simulink model "Casadi_Custom_Driver"  (R2016b)
settings: Solver=FixedStepDiscrete  StartTime=0.0  StopTime=inf  FixedStep=0.01  RelTol=1e-3  EnableMultiTasking=on
undefined symbols (not defined in the file): dimensionsFactor, DiscIntNeverNeededParam, vehicle_name, VehicleRoadInfoStructSize
libraries: simulink x39, SCANeR_API x36
(part 1 of 3)
settings Model: SimulationMode=accelerator  TunableVars=vehicle_name  TunableVarsStorageClass=ExportedGlobal  Creator=a192819  LastModifiedBy=z041288
settings DataIOCC: LimitDataPoints=on  SaveFormat=Array  SaveOutput=off  SignalLogging=off  DSMLogging=off  SaveTime=off  SignalLoggingName=virtual_driver
settings DebuggingCC: SignalInfNanChecking=warning  UnderspecifiedInitializationDetection=Classic  MergeDetectMultiDrivingBlocksExec=none  SolverPrmCheckMsg=warning  SFUnexpectedBacktrackingDiag=warning  SFNoUnconditionalDefaultTransitionDiag=warning  SFExecutionAtInitializationDiag=none
settings HardwareCC: ProdBitPerPointer=32  ProdBitPerSizeT=32  ProdBitPerPtrDiffT=32  ProdLargestAtomicFloat=None  ProdIntDivRoundTo=Undefined  ProdEndianess=Unspecified  ProdWordSize=32  ProdHWDeviceType=32-bit Generic
settings ModelReferenceCC: PropagateSignalLabelsOutOfModel=off
settings RTWCC: SystemTargetFile=grt_scanerapi.tlc  TemplateMakefile=grt_scanerapi_vc.tmf  Description=SCANeR API Real-Time Target  CustomSource=ReadConfig.c  CustomInitializer=ReadConfig();
settings STFCustomTargetCC: MatFileLogging=on  SystemTargetFile=grt_scanerapi.tlc
settings GRTTargetCC: TargetLangStandard=C89/C90 (ANSI)  ParMdlRefBuildCompliant=off  CompOptLevelCompliant=off  ConcurrentExecutionCompliant=off  CombineOutputUpdateFcns=off  CPPClassGenCompliant=off  GRTInterface=on  UseToolchainInfoCompliant=off
settings ConfigComp: CovMetricSettings=dw  CovHtmlReporting=on  CovSaveCumulativeToWorkspaceVar=on  CovSaveSingleToWorkspaceVar=on  CovExternalEMLEnable=off

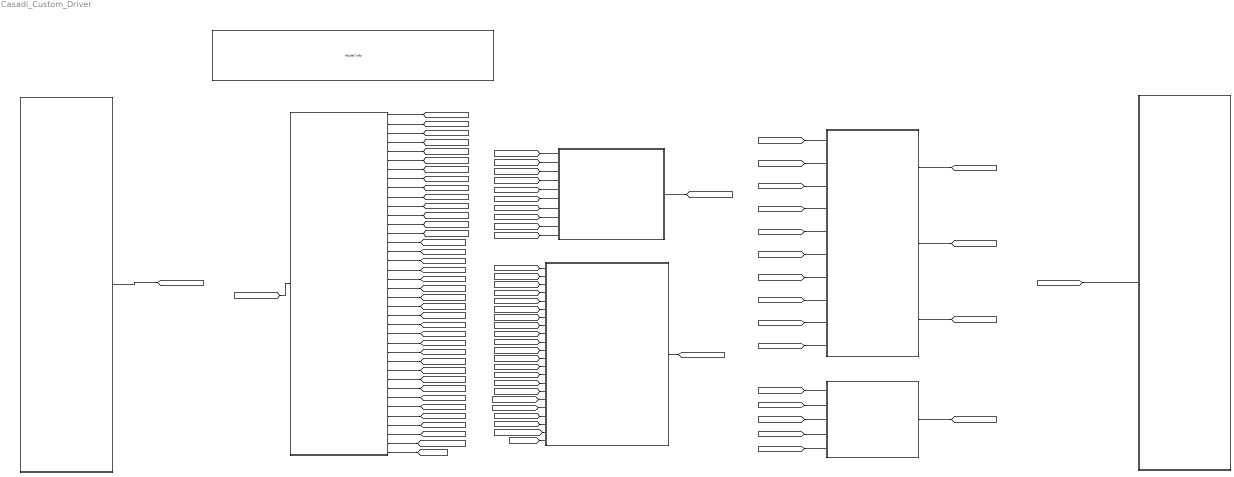
== system Casadi_Custom_Driver ==
  note: From SCANeR
  note: To SCANeR
  note: Arbitration
  note: Lateral control
  note: Longitudinal control
  note: InputSignalsManagement
  note: Custom_Driver_Architecture
  note: Custom_Driver_Environnement
  note: OutputSignalsManagement
  From Scaner : Subsystem
  Input_Signals_Management : Subsystem
  Model Info1 : simulink/Model-Wide Utilities/Model Info  Frame=on  DisplayStringWithTags=|  HorizontalTextAlignment=Left  LeftAlignmentValue=0.02  SourceBlockDiagram=Casadi_Custom_Driver  TagMaxNumber=20
      | CUSTOM DRIVER FOR SCANER
      | 
      | Developed and maintained by :
      |    - Hamid Dahmani (DEA-TDV3) (2017 => Oct. 2018)
      |    - Eric Cabrol (DEA-TDS3) (Oct. 2018 => 2020)
      |    - Eric Cabrol (DEA-TDS3) & Adithya Rajasekaran (RNTBCI) (2020 => 2021)
      |    - Eric Cabrol (DEA-TDS3), KATRE Varun-Dattakumar (RNTBCI) & Soumaya DKHEILA (DEA-TDV3) (2021 => Present)
      | 
      | Version: %<ModelVersion>
      | Last update by: %<LastModifiedBy>, Date: %<LastModificationDate>.
  Output_Signals_Management : Subsystem
  To Scaner : Subsystem
  driver manager : Subsystem
  lateral control : Subsystem
  longitudinal control : Subsystem
  wires:
  From Scaner/1(FromSCANeR_O) -> [FromSCANeR_I]
  [ToSCANeR_O] -> To Scaner/1(ToSCANeR_I)
  [FromSCANeR_I] -> Input_Signals_Management/1(From_SCANeR_I)
  Input_Signals_Management/2(vehicleHeading) -> [vehicleHeading]
  Input_Signals_Management/3(COG_Y) -> [COG_Y]
  Input_Signals_Management/4(currentSpeed) -> [currentSpeed]
  Input_Signals_Management/5(yawRate) -> [yawRate]
  Input_Signals_Management/6(currentAccel) -> [currentAcceleration]
  Input_Signals_Management/7(SteeringWheelAngle) -> [SteeringWheelAngle]
  Input_Signals_Management/8(gearEngaged) -> [gearEngaged]
  Input_Signals_Management/9(roadGap) -> [roadGap]
  Input_Signals_Management/10(roadAngle) -> [roadAngle]
  Input_Signals_Management/12(roadGapOffset) -> [roadGapOffset]
  Input_Signals_Management/11(laneGap) -> [laneGap]
  Input_Signals_Management/13(obligatorySpeed) -> [obligatorySpeed]
  Input_Signals_Management/14(obligatorySpeedState) -> [obligatorySpeedState]
  Input_Signals_Management/19(timeToReactShift) -> [timeToReactShift]
  Input_Signals_Management/16(obligatoryAccelerationState) -> [obligatoryAccelerationState]
  Input_Signals_Management/15(obligatoryAcceleration) -> [obligatoryAcceleration]
  Input_Signals_Management/17(shiftType) -> [shiftType]
  Input_Signals_Management/18(shiftValue) -> [shiftValue]
  Input_Signals_Management/27(ManualBrakeforceActivate) -> [ManualBrakeforceActivate]
  Input_Signals_Management/29(APK_Steering) -> [APK_Steering]
  Input_Signals_Management/30(clothoidAngle) -> [ClothoidAngle]
  Input_Signals_Management/28(ManualAccelActivate) -> [ManualAccelActivate]
  Input_Signals_Management/20(ManualBrakeForce) -> [ManualBrakeForce]
  Input_Signals_Management/21(ManualBrake) -> [ManualBrake]
  Input_Signals_Management/22(ManualAccel) -> [ManualAccel]
  Input_Signals_Management/25(APK_steeringActivate) -> [APK_steeringActivate]
  Input_Signals_Management/23(WantedLateralShiftSpeed) -> [WantedLateralShiftSpeed]
  Input_Signals_Management/26(ManualBrakeActivate) -> [ManualBrakeActivate]
  Input_Signals_Management/24(SteeringTorqueOrder) -> [SteeringTorqueOrder]
  Input_Signals_Management/31(SteeringTorqueRequest) -> [SteeringTorqueRequest]
  Input_Signals_Management/34(RadiusCurvatureSetPoint) -> [RadiusCurvatureSetPoint]
  Input_Signals_Management/35(VehiculeWantedGearBox) -> [VehiculeWantedGearBox]
  Input_Signals_Management/33(LaneCurvature) -> [LaneCurvature]
  Input_Signals_Management/32(DriverStatus) -> [DriverStatus]
  Input_Signals_Management/1(SCANeR_State) -> [SCANeR_State]
  [laneGap] -> lateral control/1(Lane_gap_m)
  [LaneCurvature] -> lateral control/2(RoadCurvature_pm)
  [currentSpeed] -> lateral control/3(Vh_Speed_m/s)
  [shiftValue] -> lateral control/4(Shift_Value)
  [timeToReactShift] -> lateral control/5(Shift_time_s)
  [roadAngle] -> lateral control/6(Road_Angle_rad)
  [vehicleHeading] -> lateral control/7(Vehicle_Heading_rad)
  [SCANeR_State] -> lateral control/8(SCANeR_State)
  [shiftType] -> lateral control/10(Shift_Type_1Met_0Lan)
  [roadGap] -> lateral control/11(Road_Gap_m)
  [roadGapOffset] -> lateral control/12(Road_Gap_Offset_m)
  [gearEngaged] -> lateral control/13(SCANeR_gearEngaged)
  [WantedLateralShiftSpeed] -> lateral control/14(wantedLateralShiftSpeed)
  [SteeringWheelAngle] -> lateral control/15(SW_angle_IN)
  [yawRate] -> lateral control/16(yaw rate)
  [ClothoidAngle] -> lateral control/17(clothoid_tangent_angle)
  [RadiusCurvatureSetPoint] -> lateral control/18(clothoid_flag)
  [COG_Y] -> lateral control/19(COG_Y)
  [DriverStatus] -> driver manager/2(SCANeR_DriverStatus)
  [ManualAccel] -> driver manager/3(Manual_accel_%)
  [ManualAccelActivate] -> driver manager/4(Manual_accel_%_activate)
  [ManualBrake] -> driver manager/5(Manual_brake_%)
  [ManualBrakeActivate] -> driver manager/6(Manual_brake_%_activate)
  [APK_Steering] -> driver manager/7(APK_steering_rad)
  [APK_steeringActivate] -> driver manager/8(APK_steering_rad_Activate)
  [SCANeR_State] -> driver manager/9(SCANeR_State)
  longitudinal control/1(Driver_Action_to_SCANeR_Longi) -> [Driver_Action_to_SCANeR_Longi]
  [Driver_Action_to_SCANeR_Longi] -> driver manager/1(Driver_Action_to_SCANeR_Long)
  lateral control/1(Driver_Action_to_SCANeR_Lat) -> [Driver_Action_to_SCANeR_Lat]
  [Driver_Action_to_SCANeR_Lat] -> driver manager/10(Driver_Action_to_SCANeR_Lat)
  driver manager/2(SCANeR_DriverStatus_Out) -> [DriverStatus_O]
  [DriverStatus_O] -> lateral control/9(SCANeR_DriverStatus_Out)
  driver manager/1(Driver_Action_to_SCANeR_Longi_out) -> [Driver_Action_to_SCANeR_Longi_out]
  driver manager/3(Driver_Action_to_SCANeR_Lat_out) -> [Driver_Action_to_SCANeR_Lat_out]
  Output_Signals_Management/1(ToSCANeR_O) -> [ToSCANeR_O]
  [SteeringTorqueRequest] -> Output_Signals_Management/5(SteeringTorqueRequest)
  [SteeringTorqueOrder] -> Output_Signals_Management/4(SteeringTorqueOrder)
  [VehiculeWantedGearBox] -> Output_Signals_Management/3(VehiculeWantedGearBox)
  [Driver_Action_to_SCANeR_Longi_out] -> Output_Signals_Management/1(Driver_Action_to_SCANeR_Longi_out)
  [Driver_Action_to_SCANeR_Lat_out] -> Output_Signals_Management/2(Driver_Action_to_SCANeR_Lat_out)
  [obligatorySpeed] -> longitudinal control/1(Intended_Vehicle_Speed_[m/s])
  [obligatoryAcceleration] -> longitudinal control/4(Intended_Vehicle_accel_[m/s2])
  [obligatoryAccelerationState] -> longitudinal control/6(Accel_control_on)
  [SCANeR_State] -> longitudinal control/9(SCANeR_State)
  [ManualBrakeForce] -> longitudinal control/7(Manual_braking_N)
  [currentAcceleration] -> longitudinal control/5(Vehicle_accel_[m/s2])
  [currentSpeed] -> longitudinal control/2(Vehicle_Speed_[m/s])
  [ManualBrakeforceActivate] -> longitudinal control/8(Manual_braking_Switch)
  [DriverStatus_O] -> longitudinal control/10(SCANeR_DriverStatus_Out)
  [obligatorySpeedState] -> longitudinal control/3(Speed_control_on)
  Input_Signals_Management/36(Flag_detect_banking) -> [Flag_detect_banking]
  [Flag_detect_banking] -> lateral control/20(Flag_detect_banking)
  Input_Signals_Management/37(COG_X) -> [COG_X]
  Input_Signals_Management/38(current_lateral_speed) -> [current_lateral_speed]
  [current_lateral_speed] -> lateral control/22(measured_lateral_speed)
  [COG_X] -> lateral control/21(COG_X)

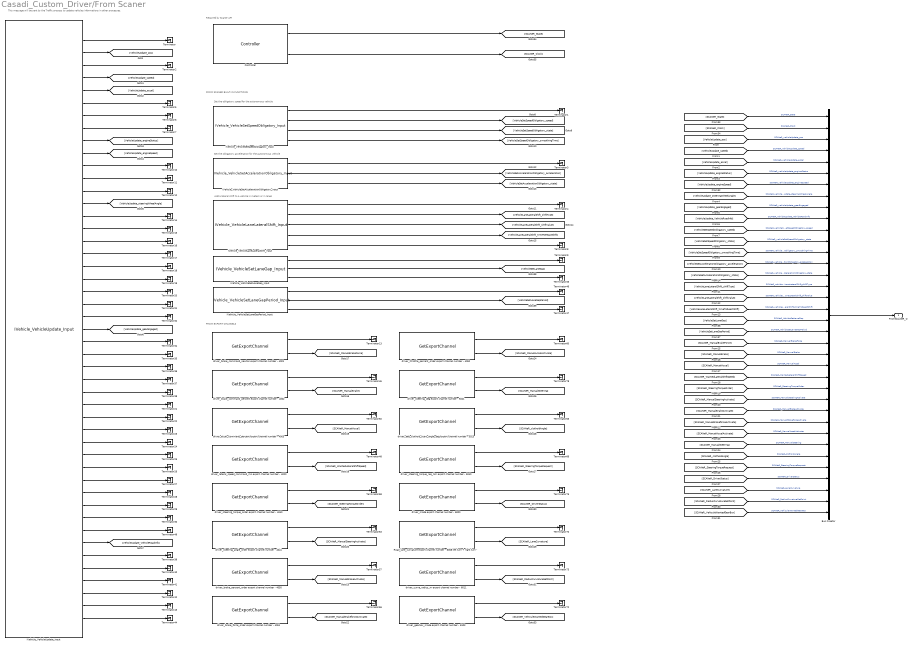
== system Casadi_Custom_Driver/From Scaner ==
  note: Set the obligatory speed for the autonomous vehicle
  note: Set the obligatory acceleration for the autonomous vehicle
  note: Add a lateral shift to a vehicle in meters or in lanes
  note: This message will be sent by the Traffic process to update vehicles informations in other processes.
  note: FROM EXPORT CHANNELS
  note: FROM SCANER BUILT-IN FUNCTIONS
  note: Required by Scaner API
  Bus Creator : BusCreator  Inputs='SCANeR_State','SCANeR_Clock','SCANeR_vehicleUpdate_pos','SCANeR_vehicleUpdate_speed','SCANeR_vehicleUpdate_accel','SCANeR_vehicleUpdate_engineStatus','SCANeR_vehicleUpdate_engineSpeed','SCANeR_vehicleUpdate_steeringWheelAngle','SCANeR_vehicleUpdate_gearEngaged','SCANeR_vehicleUpdate_VehicleRoadInfo','SCANeR_vehicleSetSpeedObligatory_speed','SCANeR_vehicleSetSpeedObligatory_state','SCANeR_vehicleSetSpeedObligatory_smoothingTime','SCANeR_vehicleSetAccelerationObligatory_acceleration','SCANeR_vehicleSetAccelerationObligatory_state','SCANeR_vehicleLaneLateralShift_shiftType','SCANeR_vehicleLaneLateralShift_shiftValue','SCANeR_vehicleLaneLateralShift_timeToReactShift','SCANeR_VehicleSetLaneGap','SCANeR_VehicleSetLaneGapPeriod','SCANeR_ManualBrakeForce','SCANeR_ManualBrake','SCANeR_ManualAccel','SCANeR_WantedLateralShiftSpeed','SCANeR_SteeringTorqueOrder','SCANeR_ManualSteeringActivate','SCANeR_ManualBrakeActivate','SCANeR_ManualBrakeforceActivate','SCANeR_ManualAccelActivate','SCANeR_ManualSteering','SCANeR_clothoidAngle','SCANeR_SteeringTorqueRequest','SCANeR_DriverStatus','SCANeR_LaneCurvature','SCANeR_RadiusCurvatureSetPoint','SCANeR_VehiculeWantedGearBox'  OutDataTypeStr=Bus: Bus_FromSCANeR
  Controller : SCANeR_API/Controller  Priority=1  Config='NEWCONFIG_Training'  ProcName='SIMULINK'  Frequency=-100  NetworkOutputFrequency=-100  TimeOut=300  IsSynchronized=on
  IVehicle_VehicleLaneLateralShift_Input : SCANeR_API/Network inputs/IVehicle/IVehicle_VehicleLaneLateralShift_Input  Priority=2  ev=off  vhlId=0
  IVehicle_VehicleSetAccelerationObligatory_Input : SCANeR_API/Network inputs/IVehicle/IVehicle_VehicleSetAccelerationObligatory_Input  Priority=2  ev=off  vhlId=0
  IVehicle_VehicleSetLaneGapPeriod_Input : SCANeR_API/Network inputs/IVehicle/IVehicle_VehicleSetLaneGapPeriod_Input  Priority=2  ev=off  vhlId=0
  IVehicle_VehicleSetLaneGap_Input : SCANeR_API/Network inputs/IVehicle/IVehicle_VehicleSetLaneGap_Input  Priority=2  ev=off  vhlId=0
  IVehicle_VehicleSetSpeedObligatory_Input : SCANeR_API/Network inputs/IVehicle/IVehicle_VehicleSetSpeedObligatory_Input  Priority=2  ev=off  vhlId=0
  IVehicle_VehicleUpdate_Input : SCANeR_API/Network inputs/IVehicle/IVehicle_VehicleUpdate_Input  Priority=2  ev=off  vhlId=0
  Road_lane_curvature export channel number - 6008 left turn + right turn - : SCANeR_API/GetExportChannel  Priority=0  ExportChannelCategory='system'  ExportChannelName='Road_lane_curvature'  VehicleId=-1
  Terminator{,1..50,53,56..58,60,63,66,70,72..73,75,78} (63 alike) : Terminator
  driver_accel_command_percent export channel number - 4003 : SCANeR_API/GetExportChannel  Priority=0  ExportChannelCategory='system'  ExportChannelName='driver_accel_command_percent'  VehicleId=-1
  driver_aeb_clothoid_start_angle_deg export channel number - 5023 : SCANeR_API/GetExportChannel  Priority=0  ExportChannelCategory='system'  ExportChannelName='driver_aeb_clothoid_start_angle_deg'  VehicleId=-1
  driver_brake_command_newton export channel number - 4001 : SCANeR_API/GetExportChannel  Priority=0  ExportChannelCategory='system'  ExportChannelName='driver_brake_command_newton'  VehicleId=-1
  driver_brake_command_percent export channel number - 4002 : SCANeR_API/GetExportChannel  Priority=0  ExportChannelCategory='system'  ExportChannelName='driver_brake_command_percent'  VehicleId=-1
  driver_brake_force_order export channel number - 4051 : SCANeR_API/GetExportChannel  Priority=0  ExportChannelCategory='system'  ExportChannelName='driver_brake_force_order'  VehicleId=-1
  driver_brake_percent_order export channel number - 4050 : SCANeR_API/GetExportChannel  Priority=0  ExportChannelCategory='system'  ExportChannelName='driver_brake_percent_order'  VehicleId=-1
  driver_curve_radius_m export channel number - 6011 : SCANeR_API/GetExportChannel  Priority=0  ExportChannelCategory='system'  ExportChannelName='driver_curve_radius_m'  VehicleId=-1
  driver_gearbox_mode export channel number - 6103 : SCANeR_API/GetExportChannel  Priority=0  ExportChannelCategory='system'  ExportChannelName='driver_gearbox_mode'  VehicleId=-1
  driver_lateral_speed_command_ms export channel number - 4020 : SCANeR_API/GetExportChannel  Priority=0  ExportChannelCategory='system'  ExportChannelName='driver_lateral_speed_command_ms'  VehicleId=-1
  driver_mode export channel number - 6000 : SCANeR_API/GetExportChannel  Priority=0  ExportChannelCategory='system'  ExportChannelName='driver_mode'  VehicleId=-1
  driver_steering_angle_order export channel number - 4041 : SCANeR_API/GetExportChannel  Priority=0  ExportChannelCategory='system'  ExportChannelName='driver_steering_angle_order'  VehicleId=-1
  driver_steering_deg export channel number - 5021 : SCANeR_API/GetExportChannel  Priority=0  ExportChannelCategory='system'  ExportChannelName='driver_steering_deg'  VehicleId=-1
  driver_steering_torque_order export channel number - 4040 : SCANeR_API/GetExportChannel  Priority=0  ExportChannelCategory='system'  ExportChannelName='driver_steering_torque_order'  VehicleId=-1
  driver_steering_torque_req_Nm export channel number - 5040 : SCANeR_API/GetExportChannel  Priority=0  ExportChannelCategory='system'  ExportChannelName='driver_steering_torque_req_Nm'  VehicleId=-1
  driver_throttle_percent_order export channel number - 4052 : SCANeR_API/GetExportChannel  Priority=0  ExportChannelCategory='system'  ExportChannelName='driver_throttle_percent_order'  VehicleId=-1
  FromSCANeR_O : Outport  OutDataTypeStr=Bus: Bus_FromSCANeR
      settings: AttributesFormatString=%<OutDataTypeStr>
  wires:
  IVehicle_VehicleUpdate_Input/1 -> Terminator/1
  IVehicle_VehicleUpdate_Input/2 -> [VehicleUpdate_pos]
  IVehicle_VehicleUpdate_Input/3 -> Terminator2/1
  IVehicle_VehicleUpdate_Input/4 -> [VehicleUpdate_speed]
  IVehicle_VehicleUpdate_Input/5 -> [VehicleUpdate_accel]
  IVehicle_VehicleUpdate_Input/6 -> Terminator5/1
  IVehicle_VehicleUpdate_Input/7 -> Terminator6/1
  IVehicle_VehicleUpdate_Input/8 -> Terminator7/1
  IVehicle_VehicleUpdate_Input/9 -> [VehicleUpdate_engineStatus]
  IVehicle_VehicleUpdate_Input/10 -> [VehicleUpdate_engineSpeed]
  IVehicle_VehicleUpdate_Input/11 -> Terminator10/1
  IVehicle_VehicleUpdate_Input/12 -> Terminator11/1
  IVehicle_VehicleUpdate_Input/13 -> Terminator12/1
  IVehicle_VehicleUpdate_Input/14 -> [VehicleUpdate_steeringWheelAngle]
  IVehicle_VehicleUpdate_Input/15 -> Terminator14/1
  IVehicle_VehicleUpdate_Input/16 -> Terminator15/1
  IVehicle_VehicleUpdate_Input/17 -> Terminator16/1
  IVehicle_VehicleUpdate_Input/18 -> Terminator17/1
  IVehicle_VehicleUpdate_Input/19 -> Terminator18/1
  IVehicle_VehicleUpdate_Input/20 -> Terminator19/1
  IVehicle_VehicleUpdate_Input/21 -> Terminator20/1
  IVehicle_VehicleUpdate_Input/22 -> Terminator31/1
  IVehicle_VehicleUpdate_Input/23 -> Terminator32/1
  IVehicle_VehicleUpdate_Input/24 -> [VehicleUpdate_gearEngaged]
  IVehicle_VehicleUpdate_Input/25 -> Terminator34/1
  IVehicle_VehicleUpdate_Input/26 -> Terminator35/1
  IVehicle_VehicleUpdate_Input/27 -> Terminator36/1
  IVehicle_VehicleUpdate_Input/28 -> Terminator37/1
  IVehicle_VehicleUpdate_Input/29 -> Terminator38/1
  IVehicle_VehicleUpdate_Input/30 -> Terminator21/1
  IVehicle_VehicleUpdate_Input/31 -> Terminator22/1
  IVehicle_VehicleUpdate_Input/32 -> Terminator23/1
  IVehicle_VehicleUpdate_Input/34 -> Terminator25/1
  IVehicle_VehicleUpdate_Input/35 -> Terminator26/1
  IVehicle_VehicleUpdate_Input/36 -> Terminator27/1
  IVehicle_VehicleUpdate_Input/37 -> Terminator28/1
  IVehicle_VehicleUpdate_Input/38 -> Terminator29/1
  IVehicle_VehicleUpdate_Input/39 -> Terminator30/1
  IVehicle_VehicleUpdate_Input/40 -> Terminator49/1
  IVehicle_VehicleUpdate_Input/41 -> [VehicleUpdate_VehicleRoadInfo]
  IVehicle_VehicleUpdate_Input/42 -> Terminator39/1
  IVehicle_VehicleUpdate_Input/43 -> Terminator40/1
  IVehicle_VehicleUpdate_Input/44 -> Terminator41/1
  IVehicle_VehicleUpdate_Input/45 -> Terminator42/1
  IVehicle_VehicleUpdate_Input/46 -> Terminator43/1
  IVehicle_VehicleUpdate_Input/47 -> Terminator44/1
  IVehicle_VehicleUpdate_Input/33 -> Terminator24/1
  IVehicle_VehicleSetSpeedObligatory_Input/1 -> Terminator1/1
  IVehicle_VehicleSetSpeedObligatory_Input/2 -> [VehicleSetSpeedObligatory_speed]
  IVehicle_VehicleSetSpeedObligatory_Input/4 -> [VehicleSetSpeedObligatory_smoothingTime]
  IVehicle_VehicleSetSpeedObligatory_Input/3 -> [VehicleSetSpeedObligatory_state]
  IVehicle_VehicleSetAccelerationObligatory_Input/1 -> Terminator3/1
  IVehicle_VehicleLaneLateralShift_Input/1 -> Terminator4/1
  IVehicle_VehicleLaneLateralShift_Input/5 -> Terminator8/1
  IVehicle_VehicleSetAccelerationObligatory_Input/2 -> [VehicleSetAccelerationObligatory_acceleration]
  IVehicle_VehicleSetAccelerationObligatory_Input/3 -> [VehicleSetAccelerationObligatory_state]
  IVehicle_VehicleLaneLateralShift_Input/2 -> [VehicleLaneLateralShift_shiftType]
  IVehicle_VehicleLaneLateralShift_Input/3 -> [VehicleLaneLateralShift_shiftValue]
  IVehicle_VehicleLaneLateralShift_Input/4 -> [VehicleLaneLateralShift_timeToReactShift]
  driver_brake_command_newton export channel number - 4001/1 -> Terminator13/1
  driver_brake_command_newton export channel number - 4001/2 -> [SCANeR_ManualBrakeForce]
  driver_brake_command_percent export channel number - 4002/1 -> Terminator45/1
  driver_brake_command_percent export channel number - 4002/2 -> [SCANeR_ManualBrake]
  driver_accel_command_percent export channel number - 4003/1 -> Terminator50/1
  driver_accel_command_percent export channel number - 4003/2 -> [SCANeR_ManualAccel]
  driver_lateral_speed_command_ms export channel number - 4020/1 -> Terminator48/1
  driver_lateral_speed_command_ms export channel number - 4020/2 -> [SCANeR_WantedLateralShiftSpeed]
  driver_steering_torque_order export channel number - 4040/1 -> Terminator58/1
  driver_steering_torque_order export channel number - 4040/2 -> [SCANeR_SteeringTorqueOrder]
  driver_steering_angle_order export channel number - 4041/1 -> Terminator53/1
  driver_steering_angle_order export channel number - 4041/2 -> [SCANeR_ManualSteeringActivate]
  driver_brake_percent_order export channel number - 4050/1 -> Terminator57/1
  driver_brake_percent_order export channel number - 4050/2 -> [SCANeR_ManualBrakeActivate]
  driver_brake_force_order export channel number - 4051/1 -> Terminator56/1
  driver_brake_force_order export channel number - 4051/2 -> [SCANeR_ManualBrakeforceActivate]
  driver_throttle_percent_order export channel number - 4052/1 -> Terminator60/1
  driver_throttle_percent_order export channel number - 4052/2 -> [SCANeR_ManualAccelActivate]
  driver_steering_deg export channel number - 5021/1 -> Terminator78/1
  driver_steering_deg export channel number - 5021/2 -> [SCANeR_ManualSteering]
  driver_aeb_clothoid_start_angle_deg export channel number - 5023/1 -> Terminator63/1
  driver_aeb_clothoid_start_angle_deg export channel number - 5023/2 -> [SCANeR_clothoidAngle]
  driver_steering_torque_req_Nm export channel number - 5040/1 -> Terminator66/1
  driver_steering_torque_req_Nm export channel number - 5040/2 -> [SCANeR_SteeringTorqueRequest]
  driver_mode export channel number - 6000/1 -> Terminator75/1
  driver_mode export channel number - 6000/2 -> [SCANeR_DriverStatus]
  Road_lane_curvature export channel number - 6008 left turn + right turn -/1 -> Terminator70/1
  Road_lane_curvature export channel number - 6008 left turn + right turn -/2 -> [SCANeR_LaneCurvature]
  driver_curve_radius_m export channel number - 6011/1 -> Terminator73/1
  driver_gearbox_mode export channel number - 6103/1 -> Terminator72/1
  driver_curve_radius_m export channel number - 6011/2 -> [SCANeR_RadiusCurvatureSetPoint]
  driver_gearbox_mode export channel number - 6103/2 -> [SCANeR_VehiculeWantedGearBox]
  [VehicleUpdate_pos] -> Bus Creator/3  "SCANeR_vehicleUpdate_pos"
  [VehicleUpdate_engineSpeed] -> Bus Creator/7  "SCANeR_vehicleUpdate_engineSpeed"
  [VehicleUpdate_engineStatus] -> Bus Creator/6  "SCANeR_vehicleUpdate_engineStatus"
  [VehicleUpdate_accel] -> Bus Creator/5  "SCANeR_vehicleUpdate_accel"
  [VehicleUpdate_speed] -> Bus Creator/4  "SCANeR_vehicleUpdate_speed"
  [VehicleUpdate_steeringWheelAngle] -> Bus Creator/8  "SCANeR_vehicleUpdate_steeringWheelAngle"
  [VehicleUpdate_gearEngaged] -> Bus Creator/9  "SCANeR_vehicleUpdate_gearEngaged"
  [VehicleUpdate_VehicleRoadInfo] -> Bus Creator/10  "SCANeR_vehicleUpdate_VehicleRoadInfo"
  [VehicleSetSpeedObligatory_speed] -> Bus Creator/11  "SCANeR_vehicleSetSpeedObligatory_speed"
  [VehicleSetSpeedObligatory_state] -> Bus Creator/12  "SCANeR_vehicleSetSpeedObligatory_state"
  [VehicleSetSpeedObligatory_smoothingTime] -> Bus Creator/13  "SCANeR_vehicleSetSpeedObligatory_smoothingTime"
  [VehicleSetAccelerationObligatory_acceleration] -> Bus Creator/14  "SCANeR_vehicleSetAccelerationObligatory_acceleration"
  [VehicleSetAccelerationObligatory_state] -> Bus Creator/15  "SCANeR_vehicleSetAccelerationObligatory_state"
  [VehicleLaneLateralShift_shiftType] -> Bus Creator/16  "SCANeR_vehicleLaneLateralShift_shiftType"
  [VehicleLaneLateralShift_shiftValue] -> Bus Creator/17  "SCANeR_vehicleLaneLateralShift_shiftValue"
  [VehicleLaneLateralShift_timeToReactShift] -> Bus Creator/18  "SCANeR_vehicleLaneLateralShift_timeToReactShift"
  Controller/1 -> [SCANeR_State]
  Controller/2 -> [SCANeR_Clock]
  [SCANeR_Clock] -> Bus Creator/2  "SCANeR_Clock"
  [SCANeR_State] -> Bus Creator/1  "SCANeR_State"
  Bus Creator/1 -> FromSCANeR_O/1
  IVehicle_VehicleSetLaneGap_Input/2 -> [VehicleSetLaneGap]
  IVehicle_VehicleSetLaneGapPeriod_Input/2 -> [VehicleSetLaneGapPeriod]
  IVehicle_VehicleSetLaneGap_Input/1 -> Terminator9/1
  IVehicle_VehicleSetLaneGap_Input/3 -> Terminator33/1
  IVehicle_VehicleSetLaneGapPeriod_Input/1 -> Terminator46/1
  IVehicle_VehicleSetLaneGapPeriod_Input/3 -> Terminator47/1
  [SCANeR_ManualBrakeForce] -> Bus Creator/21  "SCANeR_ManualBrakeForce"
  [SCANeR_ManualBrake] -> Bus Creator/22  "SCANeR_ManualBrake"
  [SCANeR_ManualAccel] -> Bus Creator/23  "SCANeR_ManualAccel"
  [SCANeR_WantedLateralShiftSpeed] -> Bus Creator/24  "SCANeR_WantedLateralShiftSpeed"
  [SCANeR_SteeringTorqueOrder] -> Bus Creator/25  "SCANeR_SteeringTorqueOrder"
  [SCANeR_ManualSteeringActivate] -> Bus Creator/26  "SCANeR_ManualSteeringActivate"
  [SCANeR_ManualBrakeActivate] -> Bus Creator/27  "SCANeR_ManualBrakeActivate"
  [SCANeR_ManualBrakeforceActivate] -> Bus Creator/28  "SCANeR_ManualBrakeforceActivate"
  [SCANeR_ManualAccelActivate] -> Bus Creator/29  "SCANeR_ManualAccelActivate"
  [SCANeR_ManualSteering] -> Bus Creator/30  "SCANeR_ManualSteering"
  [SCANeR_clothoidAngle] -> Bus Creator/31  "SCANeR_clothoidAngle"
  [SCANeR_SteeringTorqueRequest] -> Bus Creator/32  "SCANeR_SteeringTorqueRequest"
  [SCANeR_DriverStatus] -> Bus Creator/33  "SCANeR_DriverStatus"
  [SCANeR_LaneCurvature] -> Bus Creator/34  "SCANeR_LaneCurvature"
  [SCANeR_RadiusCurvatureSetPoint] -> Bus Creator/35  "SCANeR_RadiusCurvatureSetPoint"
  [SCANeR_VehiculeWantedGearBox] -> Bus Creator/36  "SCANeR_VehiculeWantedGearBox"
  [VehicleSetLaneGap] -> Bus Creator/19  "SCANeR_VehicleSetLaneGap"
  [VehicleSetLaneGapPeriod] -> Bus Creator/20  "SCANeR_VehicleSetLaneGapPeriod"

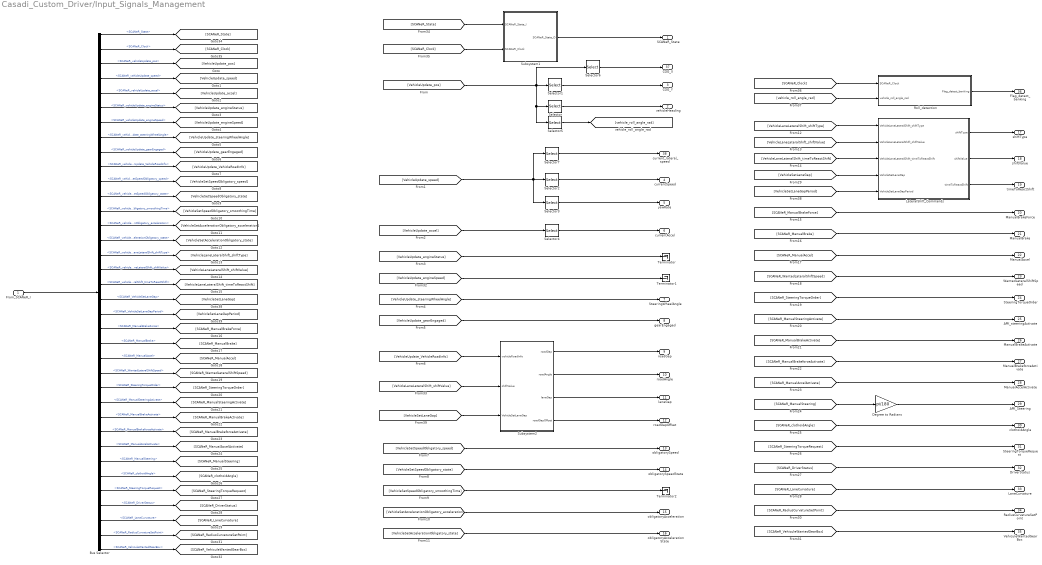
== system Casadi_Custom_Driver/Input_Signals_Management ==
  From_SCANeR_I : Inport  OutDataTypeStr=Bus: Bus_FromSCANeR
      settings: AttributesFormatString=%<OutDataTypeStr>
  Bus Selector : BusSelector  OutputSignals=SCANeR_State,SCANeR_Clock,SCANeR_vehicleUpdate_pos,SCANeR_vehicleUpdate_speed,SCANeR_vehicleUpdate_accel,SCANeR_vehicleUpdate_engineStatus,SCANeR_vehicleUpdate_engineSpeed,SCANeR_vehicleUpdate_steeringWheelAngle,SCANeR_vehicleUpdate_gearEngaged,SCANeR_vehicleUpdate_VehicleRoadInfo,SCANeR_vehicleSetSpeedObligatory_speed,SCANeR_vehicleSetSpeedObligatory_state,SCANeR_vehicleSetSpeedObligatory_smoothingTime,SCANeR_vehicleSetAccelerationObligatory_acceleration,SCANeR_vehicleSetAccelerationObligatory_state,SCANeR_vehicleLaneLateralShift_shiftType,SCANeR_vehicleLaneLateralShift_shiftValue,SCANeR_vehicleLaneLateralShift_timeToReactShift,SCANeR_VehicleSetLaneGap,SCANeR_VehicleSetLaneGapPeriod,SCANeR_ManualBrakeForce,SCANeR_ManualBrake,SCANeR_ManualAccel,SCANeR_WantedLateralShiftSpeed,SCANeR_SteeringTorqueOrder,SCANeR_ManualSteeringActivate,SCANeR_ManualBrakeActivate,SCANeR_ManualBrakeforceActivate,SCANeR_ManualAccelActivate,SCANeR_ManualSteering,SCANeR_clothoidAngle,SCANeR_SteeringTorqueRequest,SCANeR_DriverStatus,SCANeR_LaneCurvature,SCANeR_RadiusCurvatureSetPoint,SCANeR_VehiculeWantedGearBox
  Degree to Radians : Gain  Gain=pi/180
  LateralShift_Commands : Subsystem
  Roll_detection : Subsystem
  Selector : Selector  InputPortWidth=6  IndexOptions=Index vector (dialog)  Indices=[4]  OutputSizes=1
  Selector1 : Selector  InputPortWidth=6  IndexOptions=Index vector (dialog)  Indices=[2]  OutputSizes=1
  Selector2 : Selector  InputPortWidth=6  IndexOptions=Index vector (dialog)  Indices=[1]  OutputSizes=1
  Selector3 : Selector  InputPortWidth=6  IndexOptions=Index vector (dialog)  Indices=[4]  OutputSizes=1
  Selector4 : Selector  InputPortWidth=6  IndexOptions=Index vector (dialog)  Indices=[1]  OutputSizes=1
  Selector5 : Selector  InputPortWidth=6  IndexOptions=Index vector (dialog)  Indices=[6]  OutputSizes=1
  Selector6 : Selector  InputPortWidth=6  IndexOptions=Index vector (dialog)  Indices=[1]  OutputSizes=1
  Selector7 : Selector  InputPortWidth=6  IndexOptions=Index vector (dialog)  Indices=[2]  OutputSizes=1
  Subsystem1 : Subsystem
  Subsystem2 : Subsystem
  Terminator : Terminator
  Terminator1 : Terminator
  Terminator2 : Terminator
  SCANeR_State : Outport
      settings: AttributesFormatString=%<Unit>
  vehicleHeading : Outport  Port=2
      settings: AttributesFormatString=%<Unit>
  COG_Y : Outport  Port=3
      settings: AttributesFormatString=%<Unit>
  currentSpeed : Outport  Port=4
      settings: AttributesFormatString=%<Unit>
  yawRate : Outport  Port=5
      settings: AttributesFormatString=%<Unit>
  currentAccel : Outport  Port=6
      settings: AttributesFormatString=%<Unit>
  SteeringWheelAngle : Outport  Port=7
      settings: AttributesFormatString=%<Unit>
  gearEngaged : Outport  Port=8
      settings: AttributesFormatString=%<Unit>
  roadGap : Outport  Port=9
      settings: AttributesFormatString=%<Unit>
  roadAngle : Outport  Port=10
      settings: AttributesFormatString=%<Unit>
  laneGap : Outport  Port=11
      settings: AttributesFormatString=%<Unit>
  roadGapOffset : Outport  Port=12
      settings: AttributesFormatString=%<Unit>
  obligatorySpeed : Outport  Port=13
      settings: AttributesFormatString=%<Unit>
  obligatorySpeedState : Outport  Port=14
      settings: AttributesFormatString=%<Unit>
  obligatoryAcceleration : Outport  Port=15
      settings: AttributesFormatString=%<Unit>
  obligatoryAccelerationState : Outport  Port=16
      settings: AttributesFormatString=%<Unit>
  shiftType : Outport  Port=17
      settings: AttributesFormatString=%<Unit>
  shiftValue : Outport  Port=18
      settings: AttributesFormatString=%<Unit>
  timeToReactShift : Outport  Port=19
      settings: AttributesFormatString=%<Unit>
  ManualBrakeForce : Outport  Port=20
      settings: AttributesFormatString=%<Unit>
  ManualBrake : Outport  Port=21
      settings: AttributesFormatString=%<Unit>
  ManualAccel : Outport  Port=22
      settings: AttributesFormatString=%<Unit>
  WantedLateralShiftSpeed : Outport  Port=23
      settings: AttributesFormatString=%<Unit>
  SteeringTorqueOrder : Outport  Port=24
      settings: AttributesFormatString=%<Unit>
  APK_steeringActivate : Outport  Port=25
      settings: AttributesFormatString=%<Unit>
  ManualBrakeActivate : Outport  Port=26
      settings: AttributesFormatString=%<Unit>
  ManualBrakeforceActivate : Outport  Port=27
      settings: AttributesFormatString=%<Unit>
  ManualAccelActivate : Outport  Port=28
      settings: AttributesFormatString=%<Unit>
  APK_Steering : Outport  Port=29
      settings: AttributesFormatString=%<Unit>
  clothoidAngle : Outport  Port=30
      settings: AttributesFormatString=%<Unit>
  SteeringTorqueRequest : Outport  Port=31
      settings: AttributesFormatString=%<Unit>
  DriverStatus : Outport  Port=32
      settings: AttributesFormatString=%<Unit>
  LaneCurvature : Outport  Port=33
      settings: AttributesFormatString=%<Unit>
  RadiusCurvatureSetPoint : Outport  Port=34
      settings: AttributesFormatString=%<Unit>
  VehiculeWantedGearBox : Outport  Port=35
      settings: AttributesFormatString=%<Unit>
  Flag_detect_banking : Outport  Port=36
  COG_X : Outport  Port=37
  current_lateral_speed : Outport  Port=38
  wires:
  From_SCANeR_I/1 -> Bus Selector/1
  Bus Selector/36 -> [SCANeR_VehiculeWantedGearBox]  "<SCANeR_VehiculeWantedGearBox>"
  Bus Selector/35 -> [SCANeR_RadiusCurvatureSetPoint]  "<SCANeR_RadiusCurvatureSetPoint>"
  Bus Selector/34 -> [SCANeR_LaneCurvature]  "<SCANeR_LaneCurvature>"
  Bus Selector/33 -> [SCANeR_DriverStatus]  "<SCANeR_DriverStatus>"
  Bus Selector/32 -> [SCANeR_SteeringTorqueRequest]  "<SCANeR_SteeringTorqueRequest>"
  Bus Selector/31 -> [SCANeR_clothoidAngle]  "<SCANeR_clothoidAngle>"
  Bus Selector/30 -> [SCANeR_ManualSteering]  "<SCANeR_ManualSteering>"
  Bus Selector/29 -> [SCANeR_ManualAccelActivate]  "<SCANeR_ManualAccelActivate>"
  Bus Selector/28 -> [SCANeR_ManualBrakeforceActivate]  "<SCANeR_ManualBrakeforceActivate>"
  Bus Selector/27 -> [SCANeR_ManualBrakeActivate]  "<SCANeR_ManualBrakeActivate>"
  Bus Selector/26 -> [SCANeR_ManualSteeringActivate]  "<SCANeR_ManualSteeringActivate>"
  Bus Selector/25 -> [SCANeR_SteeringTorqueOrder]  "<SCANeR_SteeringTorqueOrder>"
  Bus Selector/24 -> [SCANeR_WantedLateralShiftSpeed]  "<SCANeR_WantedLateralShiftSpeed>"
  Bus Selector/23 -> [SCANeR_ManualAccel]  "<SCANeR_ManualAccel>"
  Bus Selector/22 -> [SCANeR_ManualBrake]  "<SCANeR_ManualBrake>"
  Bus Selector/21 -> [SCANeR_ManualBrakeForce]  "<SCANeR_ManualBrakeForce>"
  Bus Selector/18 -> [VehicleLaneLateralShift_timeToReactShift]  "<SCANeR_vehicleLaneLateralShift_timeToReactShift>"
  Bus Selector/17 -> [VehicleLaneLateralShift_shiftValue]  "<SCANeR_vehicleLaneLateralShift_shiftValue>"
  Bus Selector/16 -> [VehicleLaneLateralShift_shiftType]  "<SCANeR_vehicleLaneLateralShift_shiftType>"
  Bus Selector/15 -> [VehicleSetAccelerationObligatory_state]  "<SCANeR_vehicleSetAccelerationObligatory_state>"
  Bus Selector/14 -> [VehicleSetAccelerationObligatory_acceleration]  "<SCANeR_vehicleSetAccelerationObligatory_acceleration>"
  Bus Selector/13 -> [VehicleSetSpeedObligatory_smoothingTime]  "<SCANeR_vehicleSetSpeedObligatory_smoothingTime>"
  Bus Selector/12 -> [VehicleSetSpeedObligatory_state]  "<SCANeR_vehicleSetSpeedObligatory_state>"
  Bus Selector/11 -> [VehicleSetSpeedObligatory_speed]  "<SCANeR_vehicleSetSpeedObligatory_speed>"
  Bus Selector/10 -> [VehicleUpdate_VehicleRoadInfo]  "<SCANeR_vehicleUpdate_VehicleRoadInfo>"
  Bus Selector/9 -> [VehicleUpdate_gearEngaged]  "<SCANeR_vehicleUpdate_gearEngaged>"
  Bus Selector/8 -> [VehicleUpdate_steeringWheelAngle]  "<SCANeR_vehicleUpdate_steeringWheelAngle>"
  Bus Selector/7 -> [VehicleUpdate_engineSpeed]  "<SCANeR_vehicleUpdate_engineSpeed>"
  Bus Selector/6 -> [VehicleUpdate_engineStatus]  "<SCANeR_vehicleUpdate_engineStatus>"
  Bus Selector/5 -> [VehicleUpdate_accel]  "<SCANeR_vehicleUpdate_accel>"
  Bus Selector/4 -> [VehicleUpdate_speed]  "<SCANeR_vehicleUpdate_speed>"
  Bus Selector/3 -> [VehicleUpdate_pos]  "<SCANeR_vehicleUpdate_pos>"
  [VehicleUpdate_pos] -> Selector6/1, Selector1/1, Selector5/1, Selector/1
  Selector/1 -> vehicleHeading/1
  Selector1/1 -> COG_Y/1
  Selector2/1 -> currentSpeed/1
  Selector3/1 -> yawRate/1
  [VehicleUpdate_speed] -> Selector7/1, Selector3/1, Selector2/1
  Selector4/1 -> currentAccel/1
  [VehicleUpdate_accel] -> Selector4/1
  [VehicleUpdate_engineStatus] -> Terminator/1
  [VehicleUpdate_engineSpeed] -> Terminator1/1
  [VehicleUpdate_steeringWheelAngle] -> SteeringWheelAngle/1
  [VehicleUpdate_gearEngaged] -> gearEngaged/1
  [VehicleUpdate_VehicleRoadInfo] -> Subsystem2/1(vehicleRoadInfo)
  Subsystem2/1(roadGap) -> roadGap/1
  Subsystem2/2(roadAngle) -> roadAngle/1
  Subsystem2/3(laneGap) -> laneGap/1
  Subsystem2/4(roadGapOffset) -> roadGapOffset/1
  [VehicleLaneLateralShift_shiftValue] -> Subsystem2/2(shiftValue)
  [VehicleSetSpeedObligatory_speed] -> obligatorySpeed/1
  [VehicleSetSpeedObligatory_state] -> obligatorySpeedState/1
  [VehicleSetSpeedObligatory_smoothingTime] -> Terminator2/1
  [VehicleSetAccelerationObligatory_acceleration] -> obligatoryAcceleration/1
  [VehicleSetAccelerationObligatory_state] -> obligatoryAccelerationState/1
  [SCANeR_ManualBrakeForce] -> ManualBrakeForce/1
  [SCANeR_ManualBrake] -> ManualBrake/1
  [SCANeR_ManualAccel] -> ManualAccel/1
  [SCANeR_WantedLateralShiftSpeed] -> WantedLateralShiftSpeed/1
  [SCANeR_SteeringTorqueOrder] -> SteeringTorqueOrder/1
  [SCANeR_ManualSteeringActivate] -> APK_steeringActivate/1
  [SCANeR_ManualBrakeActivate] -> ManualBrakeActivate/1
  [SCANeR_ManualBrakeforceActivate] -> ManualBrakeforceActivate/1
  [SCANeR_ManualAccelActivate] -> ManualAccelActivate/1
  [SCANeR_ManualSteering] -> Degree to Radians/1
  [SCANeR_clothoidAngle] -> clothoidAngle/1
  [SCANeR_SteeringTorqueRequest] -> SteeringTorqueRequest/1
  [SCANeR_DriverStatus] -> DriverStatus/1
  [SCANeR_LaneCurvature] -> LaneCurvature/1
  [SCANeR_RadiusCurvatureSetPoint] -> RadiusCurvatureSetPoint/1
  [SCANeR_VehiculeWantedGearBox] -> VehiculeWantedGearBox/1
  Bus Selector/2 -> [SCANeR_Clock]  "<SCANeR_Clock>"
  Bus Selector/1 -> [SCANeR_State]  "<SCANeR_State>"
  [SCANeR_Clock] -> Subsystem1/2(SCANeR_Clock)
  [SCANeR_State] -> Subsystem1/1(SCANeR_State_I)
  Subsystem1/1(SCANeR_State_O) -> SCANeR_State/1
  Degree to Radians/1 -> APK_Steering/1
  Selector5/1 -> [vehicle_roll_angle_rad]
  [SCANeR_Clock] -> Roll_detection/1(SCANeR_Clock)
  [vehicle_roll_angle_rad] -> Roll_detection/2(vehicle_roll_angle_rad)
  Roll_detection/1(Flag_detect_banking) -> Flag_detect_banking/1
  Bus Selector/19 -> [VehicleSetLaneGap]  "<SCANeR_VehicleSetLaneGap>"
  Bus Selector/20 -> [VehicleSetLaneGapPeriod]  "<SCANeR_VehicleSetLaneGapPeriod>"
  [VehicleLaneLateralShift_shiftType] -> LateralShift_Commands/1(VehicleLaneLateralShift_shiftType)
  [VehicleLaneLateralShift_shiftValue] -> LateralShift_Commands/2(VehicleLaneLateralShift_shiftValue)
  [VehicleSetLaneGapPeriod] -> LateralShift_Commands/5(VehicleSetLaneGapPeriod)
  LateralShift_Commands/1(shiftType) -> shiftType/1
  LateralShift_Commands/2(shiftValue) -> shiftValue/1
  LateralShift_Commands/3(timeToReactShift) -> timeToReactShift/1
  [VehicleLaneLateralShift_timeToReactShift] -> LateralShift_Commands/3(VehicleLaneLateralShift_timeToReactShift)
  [VehicleSetLaneGap] -> LateralShift_Commands/4(VehicleSetLaneGap)
  [VehicleSetLaneGap] -> Subsystem2/3(VehicleSetLaneGap)
  Selector6/1 -> COG_X/1
  Selector7/1 -> current_lateral_speed/1

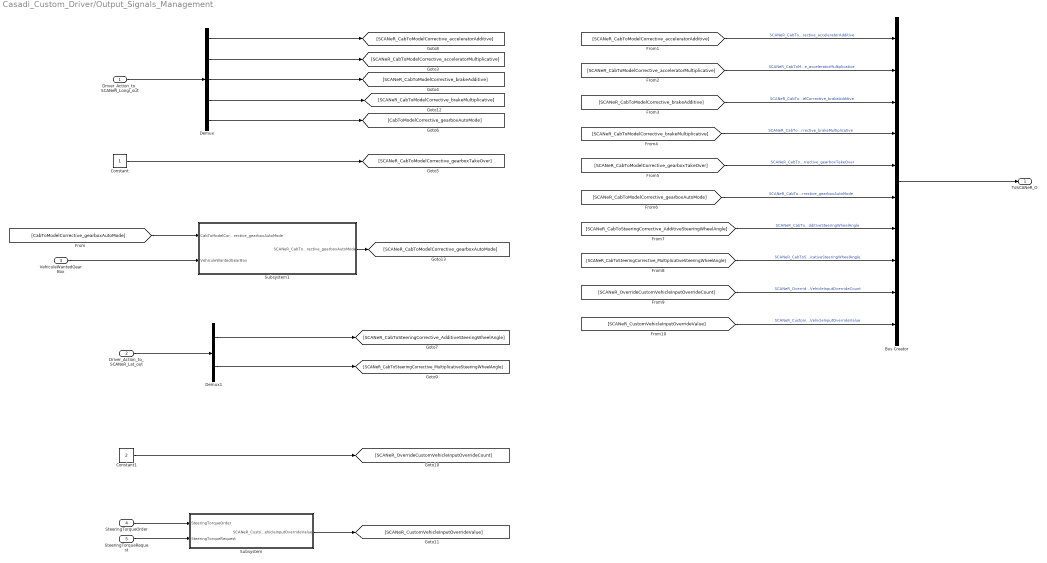
== system Casadi_Custom_Driver/Output_Signals_Management ==
  Driver_Action_to_SCANeR_Longi_out : Inport
  Driver_Action_to_SCANeR_Lat_out : Inport  Port=2
  VehiculeWantedGearBox : Inport  Port=3
  SteeringTorqueOrder : Inport  Port=4
  SteeringTorqueRequest : Inport  Port=5
  Bus Creator : BusCreator  Inputs=10
  Constant : Constant
  Constant1 : Constant  Value=2
  Demux : Demux  Outputs=5
  Demux1 : Demux  Outputs=2
  Subsystem : Subsystem
  Subsystem1 : Subsystem
  ToSCANeR_O : Outport  OutDataTypeStr=Bus: Bus_ToSCANeR
      settings: AttributesFormatString=%<OutDataTypeStr>
  wires:
  Demux/1 -> [SCANeR_CabToModelCorrective_acceleratorAdditive]
  Demux/2 -> [SCANeR_CabToModelCorrective_acceleratorMultiplicative]
  Demux/3 -> [SCANeR_CabToModelCorrective_brakeAdditive]
  Demux/4 -> [SCANeR_CabToModelCorrective_brakeMultiplicative]
  Demux/5 -> [CabToModelCorrective_gearboxAutoMode]
  Constant/1 -> [SCANeR_CabToModelCorrective_gearboxTakeOver]
  Driver_Action_to_SCANeR_Longi_out/1 -> Demux/1
  Driver_Action_to_SCANeR_Lat_out/1 -> Demux1/1
  Demux1/1 -> [SCANeR_CabToSteeringCorrective_AdditiveSteeringWheelAngle]
  Demux1/2 -> [SCANeR_CabToSteeringCorrective_MultiplicativeSteeringWheelAngle]
  Constant1/1 -> [SCANeR_OverrideCustomVehicleInputOverrideCount]
  Subsystem/1(SCANeR_CustomVehicleInputOverrideValue) -> [SCANeR_CustomVehicleInputOverrideValue]
  SteeringTorqueRequest/1 -> Subsystem/2(SteeringTorqueRequest)
  SteeringTorqueOrder/1 -> Subsystem/1(SteeringTorqueOrder)
  Bus Creator/1 -> ToSCANeR_O/1
  [SCANeR_CabToModelCorrective_acceleratorAdditive] -> Bus Creator/1  "SCANeR_CabToModelCorrective_acceleratorAdditive"
  [SCANeR_CabToModelCorrective_acceleratorMultiplicative] -> Bus Creator/2  "SCANeR_CabToModelCorrective_acceleratorMultiplicative"
  [SCANeR_CabToModelCorrective_brakeAdditive] -> Bus Creator/3  "SCANeR_CabToModelCorrective_brakeAdditive"
  [SCANeR_CabToModelCorrective_brakeMultiplicative] -> Bus Creator/4  "SCANeR_CabToModelCorrective_brakeMultiplicative"
  [SCANeR_CabToModelCorrective_gearboxTakeOver] -> Bus Creator/5  "SCANeR_CabToModelCorrective_gearboxTakeOver"
  [SCANeR_CabToModelCorrective_gearboxAutoMode] -> Bus Creator/6  "SCANeR_CabToModelCorrective_gearboxAutoMode"
  [SCANeR_OverrideCustomVehicleInputOverrideCount] -> Bus Creator/9  "SCANeR_OverrideCustomVehicleInputOverrideCount"
  [SCANeR_CabToSteeringCorrective_AdditiveSteeringWheelAngle] -> Bus Creator/7  "SCANeR_CabToSteeringCorrective_AdditiveSteeringWheelAngle"
  [SCANeR_CabToSteeringCorrective_MultiplicativeSteeringWheelAngle] -> Bus Creator/8  "SCANeR_CabToSteeringCorrective_MultiplicativeSteeringWheelAngle"
  [SCANeR_CustomVehicleInputOverrideValue] -> Bus Creator/10  "SCANeR_CustomVehicleInputOverrideValue"
  [CabToModelCorrective_gearboxAutoMode] -> Subsystem1/1(CabToModelCorrective_gearboxAutoMode)
  VehiculeWantedGearBox/1 -> Subsystem1/2(VehiculeWantedGearBox)
  Subsystem1/1(SCANeR_CabToModelCorrective_gearboxAutoMode) -> [SCANeR_CabToModelCorrective_gearboxAutoMode]

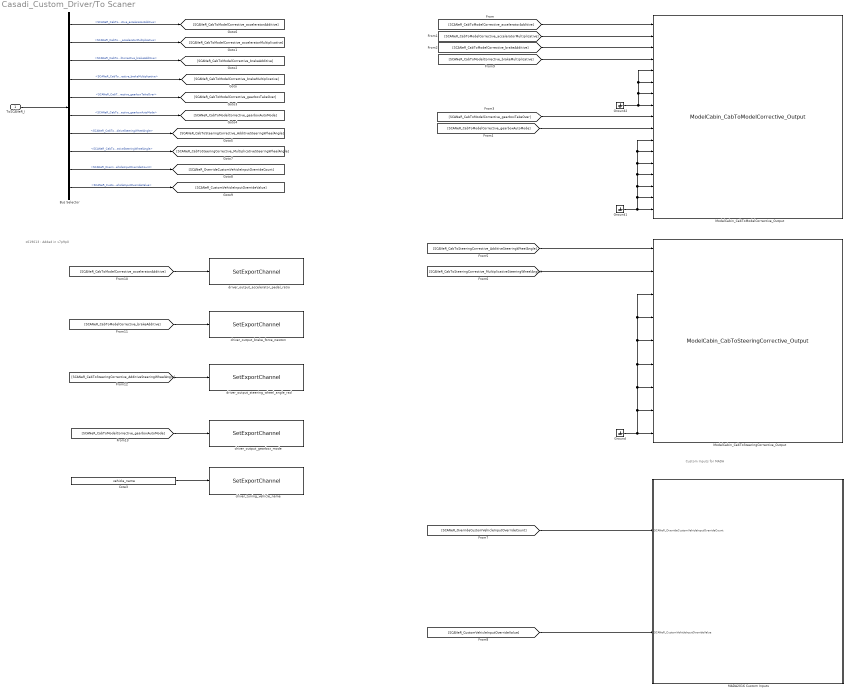
== system Casadi_Custom_Driver/To Scaner ==
  note: Custom Inputs for MADA
  note: z019013 : Added in v7p9p0
  ToSCANeR_I : Inport  OutDataTypeStr=Bus: Bus_ToSCANeR
      settings: AttributesFormatString=%<OutDataTypeStr>
  Bus Selector : BusSelector  OutputSignals=SCANeR_CabToModelCorrective_acceleratorAdditive,SCANeR_CabToModelCorrective_acceleratorMultiplicative,SCANeR_CabToModelCorrective_brakeAdditive,SCANeR_CabToModelCorrective_brakeMultiplicative,SCANeR_CabToModelCorrective_gearboxTakeOver,SCANeR_CabToModelCorrective_gearboxAutoMode,SCANeR_CabToSteeringCorrective_AdditiveSteeringWheelAngle,SCANeR_CabToSteeringCorrective_MultiplicativeSteeringWheelAngle,SCANeR_OverrideCustomVehicleInputOverrideCount,SCANeR_CustomVehicleInputOverrideValue
  Cste3 : Constant  Value=vehicle_name  SampleTime=0.01
  Ground : Ground
  Ground1 : Ground
  Ground2 : Ground
  MADA2016 Custom Inputs : Subsystem  Description=|
      | MADA_Custom_Inputs
      |
      | 0                  BrakeWheelTorqueOrder
      | 1                  Nm_BrakeWheelTorque
      | 2                  PWTWheelTorqueOrder
      | 3	Nm_PWTWheelTorque
      | 4	SteeringWheelOrder
      | 5	SteeringWheelRequest
      | 6	MODE4RD_0conf_1agil_2normal
      | 7	SWITCH4RD_1activ_0desactiv
      | 8	LKATorqueOrder
      | 9	LKATorqueRequest
      | 10	Driver_SteeringWheelTorqueOrder
      | 11	Driver_SteeringWheelTorqueRequest
      | 12	BrakePumpPrefillOrder
      mask Display: disp(sprintf(['MADA_Custom_Inputs \n']))
  ModelCabin_CabToModelCorrective_Output : SCANeR_API/SHM outputs/ModelCabin/ModelCabin_CabToModelCorrective_Output  Priority=2  shmId=0
  ModelCabin_CabToSteeringCorrective_Output : SCANeR_API/SHM outputs/ModelCabin/ModelCabin_CabToSteeringCorrective_Output  Priority=2  shmId=0
  driver_output_accelerator_pedal_ratio : SCANeR_API/SetExportChannel  Priority=0  ExportChannelCategory='system'  ExportChannelName='driver_output_accelerator_pedal_ratio'  VehicleId=-1
  driver_output_brake_force_newton : SCANeR_API/SetExportChannel  Priority=0  ExportChannelCategory='system'  ExportChannelName='driver_output_brake_force_newton'  VehicleId=-1
  driver_output_gearbox_mode : SCANeR_API/SetExportChannel  Priority=0  ExportChannelCategory='system'  ExportChannelName='driver_output_gearbox_mode'  VehicleId=-1
  driver_output_steering_wheel_angle_rad : SCANeR_API/SetExportChannel  Priority=0  ExportChannelCategory='system'  ExportChannelName='driver_output_steering_wheel_angle_rad'  VehicleId=-1
  driver_tuning_vehicle_name : SCANeR_API/SetExportChannel  Priority=0  ExportChannelCategory='system'  ExportChannelName='driver_tuning_vehicle_name'  VehicleId=-1
  wires:
  Ground1/1 -> ModelCabin_CabToModelCorrective_Output/17, ModelCabin_CabToModelCorrective_Output/16, ModelCabin_CabToModelCorrective_Output/15, ModelCabin_CabToModelCorrective_Output/14, ModelCabin_CabToModelCorrective_Output/13, ModelCabin_CabToModelCorrective_Output/12, ModelCabin_CabToModelCorrective_Output/11
  Ground/1 -> ModelCabin_CabToSteeringCorrective_Output/9, ModelCabin_CabToSteeringCorrective_Output/8, ModelCabin_CabToSteeringCorrective_Output/7, ModelCabin_CabToSteeringCorrective_Output/6, ModelCabin_CabToSteeringCorrective_Output/5, ModelCabin_CabToSteeringCorrective_Output/4, ModelCabin_CabToSteeringCorrective_Output/3
  Ground2/1 -> ModelCabin_CabToModelCorrective_Output/8, ModelCabin_CabToModelCorrective_Output/7, ModelCabin_CabToModelCorrective_Output/6, ModelCabin_CabToModelCorrective_Output/5
  [SCANeR_OverrideCustomVehicleInputOverrideCount] -> MADA2016 Custom Inputs/1(SCANeR_OverrideCustomVehicleInputOverrideCount)
  [SCANeR_CustomVehicleInputOverrideValue] -> MADA2016 Custom Inputs/2(SCANeR_CustomVehicleInputOverrideValue)
  [SCANeR_CabToModelCorrective_acceleratorAdditive] -> ModelCabin_CabToModelCorrective_Output/1
  [SCANeR_CabToModelCorrective_acceleratorMultiplicative] -> ModelCabin_CabToModelCorrective_Output/2
  [SCANeR_CabToModelCorrective_brakeAdditive] -> ModelCabin_CabToModelCorrective_Output/3
  [SCANeR_CabToModelCorrective_gearboxTakeOver] -> ModelCabin_CabToModelCorrective_Output/9
  [SCANeR_CabToModelCorrective_gearboxAutoMode] -> ModelCabin_CabToModelCorrective_Output/10
  [SCANeR_CabToSteeringCorrective_AdditiveSteeringWheelAngle] -> ModelCabin_CabToSteeringCorrective_Output/1
  [SCANeR_CabToSteeringCorrective_MultiplicativeSteeringWheelAngle] -> ModelCabin_CabToSteeringCorrective_Output/2
  [SCANeR_CabToModelCorrective_brakeMultiplicative] -> ModelCabin_CabToModelCorrective_Output/4
  ToSCANeR_I/1 -> Bus Selector/1
  Bus Selector/1 -> [SCANeR_CabToModelCorrective_acceleratorAdditive]  "<SCANeR_CabToModelCorrective_acceleratorAdditive>"
  Bus Selector/2 -> [SCANeR_CabToModelCorrective_acceleratorMultiplicative]  "<SCANeR_CabToModelCorrective_acceleratorMultiplicative>"
  Bus Selector/3 -> [SCANeR_CabToModelCorrective_brakeAdditive]  "<SCANeR_CabToModelCorrective_brakeAdditive>"
  Bus Selector/4 -> [SCANeR_CabToModelCorrective_brakeMultiplicative]  "<SCANeR_CabToModelCorrective_brakeMultiplicative>"
  Bus Selector/9 -> [SCANeR_OverrideCustomVehicleInputOverrideCount]  "<SCANeR_OverrideCustomVehicleInputOverrideCount>"
  Bus Selector/5 -> [SCANeR_CabToModelCorrective_gearboxTakeOver]  "<SCANeR_CabToModelCorrective_gearboxTakeOver>"
  Bus Selector/8 -> [SCANeR_CabToSteeringCorrective_MultiplicativeSteeringWheelAngle]  "<SCANeR_CabToSteeringCorrective_MultiplicativeSteeringWheelAngle>"
  Bus Selector/6 -> [SCANeR_CabToModelCorrective_gearboxAutoMode]  "<SCANeR_CabToModelCorrective_gearboxAutoMode>"
  Bus Selector/7 -> [SCANeR_CabToSteeringCorrective_AdditiveSteeringWheelAngle]  "<SCANeR_CabToSteeringCorrective_AdditiveSteeringWheelAngle>"
  Bus Selector/10 -> [SCANeR_CustomVehicleInputOverrideValue]  "<SCANeR_CustomVehicleInputOverrideValue>"
  [SCANeR_CabToModelCorrective_acceleratorAdditive] -> driver_output_accelerator_pedal_ratio/1
  [SCANeR_CabToModelCorrective_brakeAdditive] -> driver_output_brake_force_newton/1
  [SCANeR_CabToSteeringCorrective_AdditiveSteeringWheelAngle] -> driver_output_steering_wheel_angle_rad/1
  [SCANeR_CabToModelCorrective_gearboxAutoMode] -> driver_output_gearbox_mode/1
  Cste3/1 -> driver_tuning_vehicle_name/1

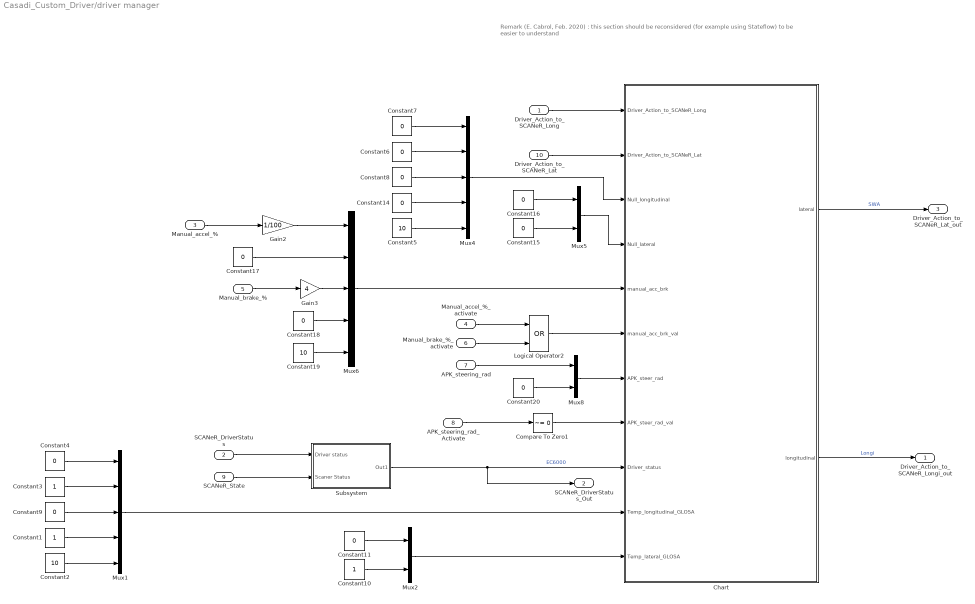
== system Casadi_Custom_Driver/driver manager ==
  note: Remark (E. Cabrol, Feb. 2020) :
      | this section should be reconsidered (for example using Stateflow) to be easier to understand
  Driver_Action_to_SCANeR_Long : Inport
  SCANeR_DriverStatus : Inport  Port=2
  Manual_accel_% : Inport  Port=3
  Manual_accel_%_activate : Inport  Port=4
  Manual_brake_% : Inport  Port=5
  Manual_brake_%_activate : Inport  Port=6
  APK_steering_rad : Inport  Port=7
  APK_steering_rad_Activate : Inport  Port=8
  SCANeR_State : Inport  Port=9
  Driver_Action_to_SCANeR_Lat : Inport  Port=10
  Chart : Stateflow chart  TreatAsAtomicUnit=on
  Compare To Zero1 : simulink/Logic and Bit Operations/Compare To Zero  relop=~=  OutDataTypeStr=boolean
  Constant1 : Constant
  Constant10 : Constant
  Constant{4,6..9,11,14..18,20} (12 alike) : Constant  Value=0
  Constant19 : Constant  Value=10
  Constant2 : Constant  Value=10
  Constant3 : Constant
  Constant5 : Constant  Value=10
  Gain2 : Gain  Gain=1/100
  Gain3 : Gain  Gain=4
  Logical Operator2 : Logic  Operator=OR  AllPortsSameDT=off  OutDataTypeStr=boolean
  Mux1 : Mux  Inputs=5
  Mux2 : Mux  Inputs=2
  Mux4 : Mux  Inputs=5
  Mux5 : Mux  Inputs=2
  Mux6 : Mux  Inputs=5
  Mux8 : Mux  Inputs=2
  Subsystem : Subsystem
  Driver_Action_to_SCANeR_Longi_out : Outport
  SCANeR_DriverStatus_Out : Outport  Port=2
  Driver_Action_to_SCANeR_Lat_out : Outport  Port=3
  wires:
  Driver_Action_to_SCANeR_Long/1 -> Chart/1(Driver_Action_to_SCANeR_Long)
  Subsystem/1(Out1) -> SCANeR_DriverStatus_Out/1, Chart/9(Driver_status)  "EC6000"
  Driver_Action_to_SCANeR_Lat/1 -> Chart/2(Driver_Action_to_SCANeR_Lat)
  Constant7/1 -> Mux4/1
  Constant14/1 -> Mux4/4
  Constant6/1 -> Mux4/2
  Constant8/1 -> Mux4/3
  Constant5/1 -> Mux4/5
  Constant15/1 -> Mux5/2
  Constant16/1 -> Mux5/1
  Mux5/1 -> Chart/4(Null_lateral)
  Mux4/1 -> Chart/3(Null_longitudinal)
  Manual_brake_%/1 -> Gain3/1
  Mux6/1 -> Chart/5(manual_acc_brk)
  Manual_accel_%/1 -> Gain2/1
  Gain2/1 -> Mux6/1
  Gain3/1 -> Mux6/3
  Logical Operator2/1 -> Chart/6(manual_acc_brk_val)
  Constant17/1 -> Mux6/2
  Constant18/1 -> Mux6/4
  Constant19/1 -> Mux6/5
  Constant20/1 -> Mux8/2
  Mux8/1 -> Chart/7(APK_steer_rad)
  Compare To Zero1/1 -> Chart/8(APK_steer_rad_val)
  Chart/1(lateral) -> Driver_Action_to_SCANeR_Lat_out/1  "SWA"
  Chart/2(longitudinal) -> Driver_Action_to_SCANeR_Longi_out/1  "Longi"
  SCANeR_DriverStatus/1 -> Subsystem/1(Driver status)
  SCANeR_State/1 -> Subsystem/2(Scaner Status)
  APK_steering_rad/1 -> Mux8/1
  APK_steering_rad_Activate/1 -> Compare To Zero1/1
  Manual_accel_%_activate/1 -> Logical Operator2/1
  Manual_brake_%_activate/1 -> Logical Operator2/2
  Constant4/1 -> Mux1/1
  Constant1/1 -> Mux1/4
  Constant3/1 -> Mux1/2
  Constant9/1 -> Mux1/3
  Constant2/1 -> Mux1/5
  Mux1/1 -> Chart/10(Temp_longitudinal_GLOSA)
  Constant10/1 -> Mux2/2
  Constant11/1 -> Mux2/1
  Mux2/1 -> Chart/11(Temp_lateral_GLOSA)
